simulink model "sample2"  (R2018b)
settings: Solver=VariableStepAuto  StartTime=0.0  StopTime=10.0  RelTol=1e-3
libraries: fl_lib x6, nesl_utility x1
settings Model: Creator=willr  LastModifiedBy=willr

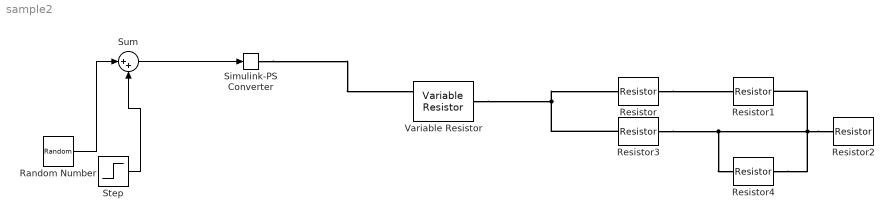
== system sample2 ==
  Random Number : RandomNumber  SampleTime=0.1
  Resistor{,1..4} (5 alike) : fl_lib/Electrical/Electrical Elements/Resistor  R=1 Ohm  i_specify=off  i_priority=None  i=0 A  i_nominal_specify=off  i_nominal_unit=A  i_nominal_value=1  v_specify=off  v_priority=None  v=0 V  v_nominal_specify=off  v_nominal_unit=V  v_nominal_value=1
  Simulink-PS Converter : nesl_utility/Simulink-PS Converter  PhysicalDomain=network_engine_domain  SubClassName=ps_input  LeftPortType=input  RightPortType=output  PseudoPeriodic=off  Frequencies=[]  NoiseDistribution=none  NoiseParameters=[]  Unit=1  AffineConversion=off  FilteringAndDerivatives=provide  SimscapeFilterOrder=1  InputFilterTimeConstant=0.001  UdotUserProvided=0
  Step : Step  SampleTime=0
  Sum : Sum  Inputs=|++
  Variable Resistor : fl_lib/Electrical/Electrical Elements/Variable Resistor  Rmin=0 Ohm  i_specify=off  i_priority=None  i=0 A  i_nominal_specify=off  i_nominal_unit=A  i_nominal_value=1  v_specify=off  v_priority=None  v=0 V  v_nominal_specify=off  v_nominal_unit=V  v_nominal_value=1
  wires:
  Random Number/1 -> Sum/1
  Step/1 -> Sum/2
  Sum/1 -> Simulink-PS Converter/1
  connections:
  Simulink-PS Converter/RConn1 -- Variable Resistor/LConn1
  Resistor2/LConn1 -- Resistor1/RConn1 -- Resistor4/RConn1 -- Resistor4/LConn1 -- Resistor3/RConn1
  Resistor/RConn1 -- Resistor1/LConn1
  Resistor3/LConn1 -- Variable Resistor/RConn1 -- Resistor/LConn1
